simulink model "exp2_obstavoid"  (R2022a)
settings: Solver=VariableStepAuto  StartTime=0.0  StopTime=20.0  RelTol=1e-3
libraries: slpidlib x3, slctrlblks x1
settings Model: Creator=Utente  LastModifiedBy=Utente

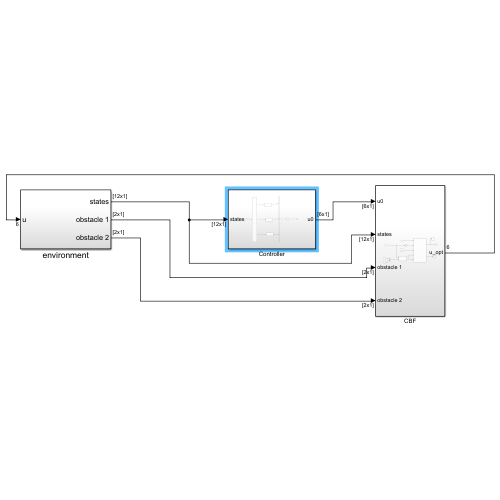
[thumbnail: Simulink's stored preview of the top-level diagram]
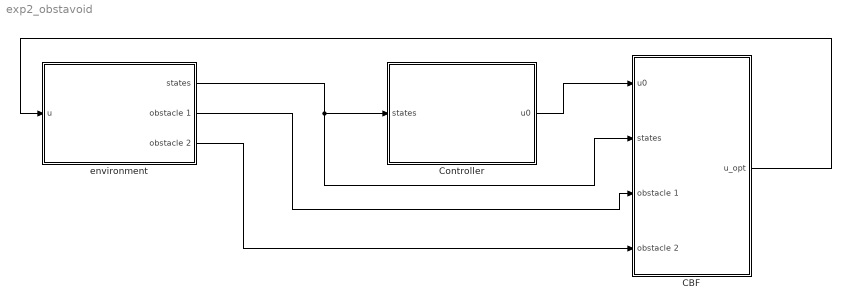
== system exp2_obstavoid ==
  CBF : Subsystem
  Controller : Subsystem
  environment : Subsystem
  wires:
  Controller/1(u0) -> CBF/1(u0)
  environment/1(states) -> CBF/2(states), Controller/1(states)
  CBF/1(u_opt) -> environment/1(u)
  environment/2(obstacle 1) -> CBF/3(obstacle 1)
  environment/3(obstacle 2) -> CBF/4(obstacle 2)

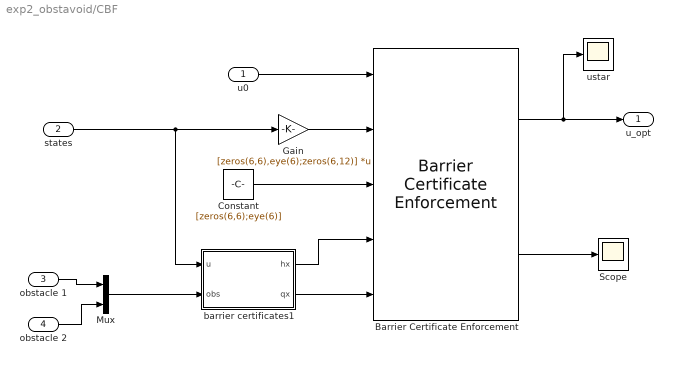
== system exp2_obstavoid/CBF ==
  u0 : Inport
  states : Inport  Port=2
  obstacle 1 : Inport  Port=3
  obstacle 2 : Inport  Port=4
  Barrier Certificate Enforcement : slctrlblks/Barrier Certificate Enforcement  nx=12  nu=6  nc=9  gamma=0.05  beta=3  external_umax=off  external_umin=off  Ts=0.1  maxiter=200  tol=1e-6  output_exitflag=on
      settings: SourceProductBaseCode=SD
  Constant : Constant  Value=[zeros(6,6);eye(6)]
  Gain : Gain  Gain=[zeros(6,6),eye(6);zeros(6,12)]  Multiplication=Matrix(K*u)
  Mux : Mux  Inputs=2
  Scope : Scope
  barrier certificates1 : MATLAB Function  TreatAsAtomicUnit=on
  ustar : Scope
  u_opt : Outport
  wires:
  Barrier Certificate Enforcement/2 -> Scope/1
  Constant/1 -> Barrier Certificate Enforcement/3
  u0/1 -> Barrier Certificate Enforcement/1
  Gain/1 -> Barrier Certificate Enforcement/2
  states/1 -> barrier certificates1/1(u), Gain/1
  Barrier Certificate Enforcement/1 -> ustar/1, u_opt/1
  barrier certificates1/1(hx) -> Barrier Certificate Enforcement/4
  barrier certificates1/2(qx) -> Barrier Certificate Enforcement/5
  obstacle 2/1 -> Mux/2
  obstacle 1/1 -> Mux/1
  Mux/1 -> barrier certificates1/2(obs)

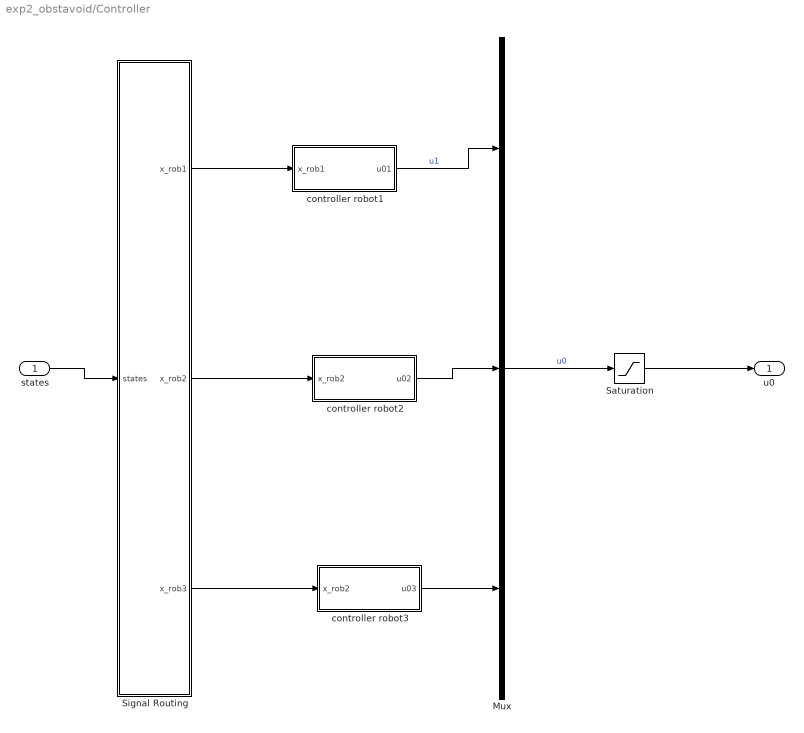
== system exp2_obstavoid/Controller ==
  states : Inport
  Mux : Mux  Inputs=3
  Saturation : Saturate  UpperLimit=10  LowerLimit=-10
  Signal Routing : MATLAB Function  TreatAsAtomicUnit=on
  controller robot1 : Subsystem
  controller robot2 : Subsystem
  controller robot3 : Subsystem
  u0 : Outport
  wires:
  states/1 -> Signal Routing/1(states)
  Signal Routing/1(x_rob1) -> controller robot1/1(x_rob1)
  Signal Routing/2(x_rob2) -> controller robot2/1(x_rob2)
  Signal Routing/3(x_rob3) -> controller robot3/1(x_rob2)
  controller robot1/1(u01) -> Mux/1  "u1"
  controller robot2/1(u02) -> Mux/2
  controller robot3/1(u03) -> Mux/3
  Mux/1 -> Saturation/1  "u0"
  Saturation/1 -> u0/1

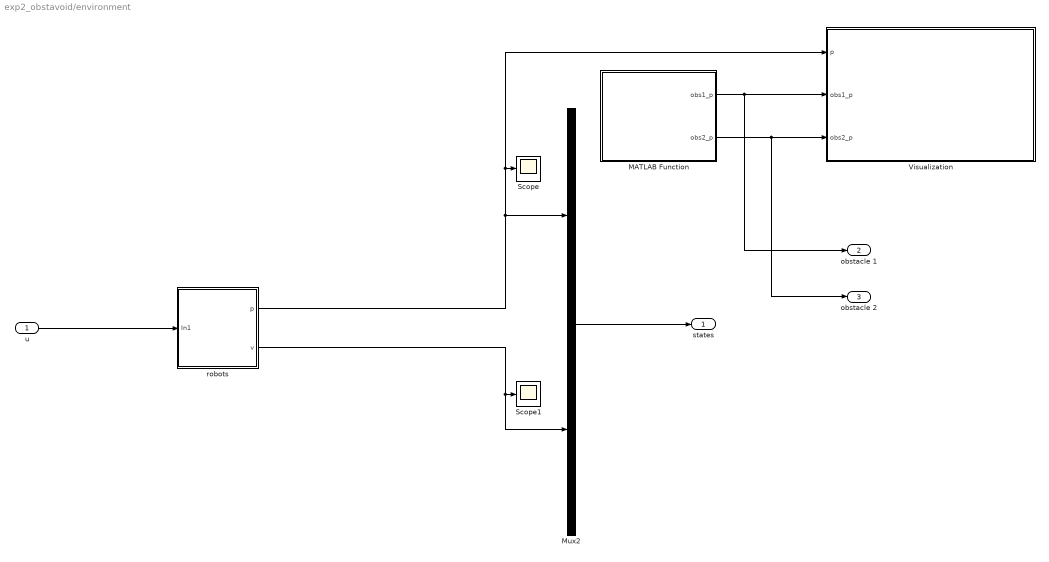
== system exp2_obstavoid/environment ==
  u : Inport
  MATLAB Function : MATLAB Function  TreatAsAtomicUnit=on
  Mux2 : Mux  Inputs=2
  Scope : Scope
  Scope1 : Scope
  Visualization : Subsystem
  robots : Subsystem
  states : Outport
  obstacle 1 : Outport  Port=2
  obstacle 2 : Outport  Port=3
  wires:
  Mux2/1 -> states/1
  robots/2(v) -> Mux2/2, Scope1/1
  robots/1(p) -> Scope/1, Visualization/1(p), Mux2/1
  u/1 -> robots/1(In1)
  MATLAB Function/1(obs1_p) -> obstacle 1/1, Visualization/2(obs1_p)
  MATLAB Function/2(obs2_p) -> obstacle 2/1, Visualization/3(obs2_p)

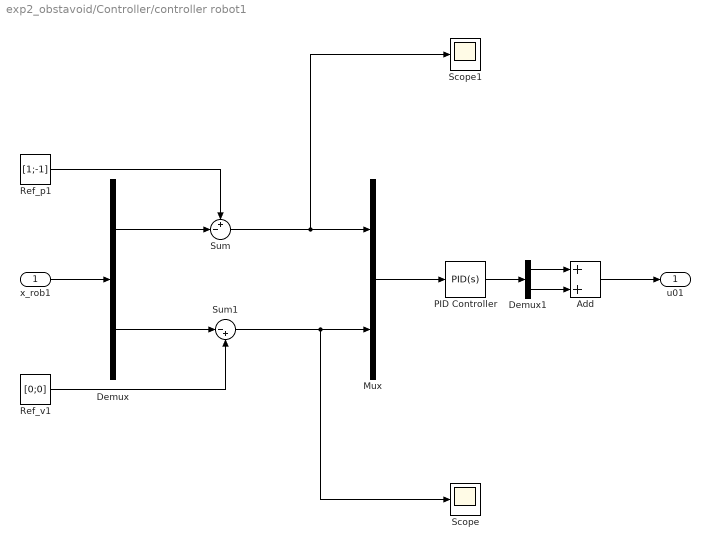
== system exp2_obstavoid/Controller/controller robot1 ==
  x_rob1 : Inport
  Add : Sum
  Demux : Demux  Outputs=2
  Demux1 : Demux  Outputs=2
  Mux : Mux  Inputs=2
  PID Controller : slpidlib/PID Controller  Controller=PID  Form=Parallel  TimeDomain=Continuous-time  UseExternalTs=off  SampleTime=-1  IntegratorMethod=Forward Euler  FilterMethod=Forward Euler  ControllerParametersSource=internal  P=5  I=0  UseKiTs=off  D=0  N=100  UseFilter=on  TunerSelectOption=Transfer Function Based (PID Tuner App)  InitialConditionSource=internal  InitialConditionForIntegrator=0  InitialConditionForFilter=0  DifferentiatorICPrevScaledInput=0  ExternalReset=none  TrackingMode=off  Kt=1  LimitOutput=off  SatLimitsSource=internal  UpperSaturationLimit=inf  LowerSaturationLimit=-inf  LinearizeAsGain=on  AntiWindupMode=none  Kb=1  POutMin=[]  POutMax=[]  IOutMin=[]  IOutMax=[]  DOutMin=[]  DOutMax=[]  NOutMin=[]  NOutMax=[]  SumOutMin=[]  SumOutMax=[]  SaturationOutMin=[]  SaturationOutMax=[]  PParamMin=[]  PParamMax=[]  IParamMin=[]  IParamMax=[]  DParamMin=[]  DParamMax=[]  NParamMin=[]  NParamMax=[]  KbParamMin=[]  KbParamMax=[]  KtParamMin=[]  KtParamMax=[]  KbOutMin=[]  KbOutMax=[]  KtOutMin=[]  KtOutMax=[]  IntegratorOutMin=[]  IntegratorOutMax=[]  FilterOutMin=[]  FilterOutMax=[]  SumI1OutMin=[]  SumI1OutMax=[]  SumI2OutMin=[]  SumI2OutMax=[]  SumI3OutMin=[]  SumI3OutMax=[]  SumI4OutMin=[]  SumI4OutMax=[]  SumDOutMin=[]  SumDOutMax=[]  DifferentiatorOutMin=[]  DifferentiatorOutMax=[]  FilterDiffOutCoefMin=[]  FilterDiffOutCoefMax=[]  ReciprocalOutMin=[]  ReciprocalOutMax=[]  SumDenOutMin=[]  SumDenOutMax=[]  SumNumOutMin=[]  SumNumOutMax=[]  DivideOutMin=[]  DivideOutMax=[]  UdiffTsProdOutMin=[]  UdiffTsProdOutMax=[]  NTsProdOutMin=[]  NTsProdOutMax=[]  UintegralTsProdOutMin=[]  UintegralTsProdOutMax=[]  UngainTsProdOutMin=[]  UngainTsProdOutMax=[]  IntegratorContinuousStateAttributes=''  IntegratorStateMustResolveToSignalObject=off  IntegratorRTWStateStorageClass=Auto  FilterContinuousStateAttributes=''  FilterStateMustResolveToSignalObject=off  FilterRTWStateStorageClass=Auto  ParallelPVariant=InternalParameters  IdealPVariant=Disabled  IVariant=InternalParameters  DVariant=InternalParameters  IntegratorVariant=Continuous  SatVariant=Disabled  AWVariant=Passthrough  PCopyVariant=Disabled  TRVariant=Disabled  FdbkBlocksVariant=Forward  IdealPFdbkVariant=Disabled  SatFdbkVariant=Disabled  DerivativeFilterVariant=ContFilter  NVariant=InternalParameters  NCopyVariant=Disabled  FilterICVariant=InternalICsFilter  IntegratorICVariant=InternalICs  ExternalResetVariant=Disabled  TRSumVariant=Passthrough  SumFdbkVariant=Disabled  SumVariant=Sum_PID  TsampFilterVariant=InternalTs  TsampNgainVariant=Passthrough  TsampIntegralVariant=Passthrough  ExternalSaturationOutDataTypeStr=Inherit: Same as second input  aMode=0
  Ref_p1 : Constant  Value=[1;-1]  VectorParams1D=off
  Ref_v1 : Constant  Value=[0;0]  VectorParams1D=off
  Scope : Scope
  Scope1 : Scope
  Sum : Sum  Inputs=+-|
  Sum1 : Sum  Inputs=|-+
  u01 : Outport
  wires:
  x_rob1/1 -> Demux/1
  Demux/1 -> Sum/2
  Ref_p1/1 -> Sum/1
  Demux/2 -> Sum1/1
  Ref_v1/1 -> Sum1/2
  Sum/1 -> Mux/1, Scope1/1
  Sum1/1 -> Mux/2, Scope/1
  Mux/1 -> PID Controller/1
  PID Controller/1 -> Demux1/1
  Demux1/2 -> Add/2
  Demux1/1 -> Add/1
  Add/1 -> u01/1

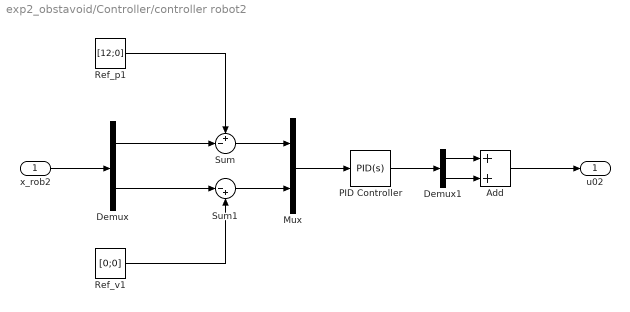
== system exp2_obstavoid/Controller/controller robot2 ==
  x_rob2 : Inport
  Add : Sum
  Demux : Demux  Outputs=2
  Demux1 : Demux  Outputs=2
  Mux : Mux  Inputs=2
  PID Controller : slpidlib/PID Controller  Controller=PID  Form=Parallel  TimeDomain=Continuous-time  UseExternalTs=off  SampleTime=-1  IntegratorMethod=Forward Euler  FilterMethod=Forward Euler  ControllerParametersSource=internal  P=5  I=0  UseKiTs=off  D=0  N=100  UseFilter=on  TunerSelectOption=Transfer Function Based (PID Tuner App)  InitialConditionSource=internal  InitialConditionForIntegrator=0  InitialConditionForFilter=0  DifferentiatorICPrevScaledInput=0  ExternalReset=none  TrackingMode=off  Kt=1  LimitOutput=off  SatLimitsSource=internal  UpperSaturationLimit=inf  LowerSaturationLimit=-inf  LinearizeAsGain=on  AntiWindupMode=none  Kb=1  POutMin=[]  POutMax=[]  IOutMin=[]  IOutMax=[]  DOutMin=[]  DOutMax=[]  NOutMin=[]  NOutMax=[]  SumOutMin=[]  SumOutMax=[]  SaturationOutMin=[]  SaturationOutMax=[]  PParamMin=[]  PParamMax=[]  IParamMin=[]  IParamMax=[]  DParamMin=[]  DParamMax=[]  NParamMin=[]  NParamMax=[]  KbParamMin=[]  KbParamMax=[]  KtParamMin=[]  KtParamMax=[]  KbOutMin=[]  KbOutMax=[]  KtOutMin=[]  KtOutMax=[]  IntegratorOutMin=[]  IntegratorOutMax=[]  FilterOutMin=[]  FilterOutMax=[]  SumI1OutMin=[]  SumI1OutMax=[]  SumI2OutMin=[]  SumI2OutMax=[]  SumI3OutMin=[]  SumI3OutMax=[]  SumI4OutMin=[]  SumI4OutMax=[]  SumDOutMin=[]  SumDOutMax=[]  DifferentiatorOutMin=[]  DifferentiatorOutMax=[]  FilterDiffOutCoefMin=[]  FilterDiffOutCoefMax=[]  ReciprocalOutMin=[]  ReciprocalOutMax=[]  SumDenOutMin=[]  SumDenOutMax=[]  SumNumOutMin=[]  SumNumOutMax=[]  DivideOutMin=[]  DivideOutMax=[]  UdiffTsProdOutMin=[]  UdiffTsProdOutMax=[]  NTsProdOutMin=[]  NTsProdOutMax=[]  UintegralTsProdOutMin=[]  UintegralTsProdOutMax=[]  UngainTsProdOutMin=[]  UngainTsProdOutMax=[]  IntegratorContinuousStateAttributes=''  IntegratorStateMustResolveToSignalObject=off  IntegratorRTWStateStorageClass=Auto  FilterContinuousStateAttributes=''  FilterStateMustResolveToSignalObject=off  FilterRTWStateStorageClass=Auto  ParallelPVariant=InternalParameters  IdealPVariant=Disabled  IVariant=InternalParameters  DVariant=InternalParameters  IntegratorVariant=Continuous  SatVariant=Disabled  AWVariant=Passthrough  PCopyVariant=Disabled  TRVariant=Disabled  FdbkBlocksVariant=Forward  IdealPFdbkVariant=Disabled  SatFdbkVariant=Disabled  DerivativeFilterVariant=ContFilter  NVariant=InternalParameters  NCopyVariant=Disabled  FilterICVariant=InternalICsFilter  IntegratorICVariant=InternalICs  ExternalResetVariant=Disabled  TRSumVariant=Passthrough  SumFdbkVariant=Disabled  SumVariant=Sum_PID  TsampFilterVariant=InternalTs  TsampNgainVariant=Passthrough  TsampIntegralVariant=Passthrough  ExternalSaturationOutDataTypeStr=Inherit: Same as second input  aMode=0
  Ref_p1 : Constant  Value=[12;0]  VectorParams1D=off
  Ref_v1 : Constant  Value=[0;0]  VectorParams1D=off
  Sum : Sum  Inputs=+-|
  Sum1 : Sum  Inputs=|-+
  u02 : Outport
  wires:
  x_rob2/1 -> Demux/1
  Demux/1 -> Sum/2
  Ref_p1/1 -> Sum/1
  Demux/2 -> Sum1/1
  Ref_v1/1 -> Sum1/2
  Add/1 -> u02/1
  Demux1/2 -> Add/2
  Mux/1 -> PID Controller/1
  Sum/1 -> Mux/1
  Sum1/1 -> Mux/2
  PID Controller/1 -> Demux1/1
  Demux1/1 -> Add/1

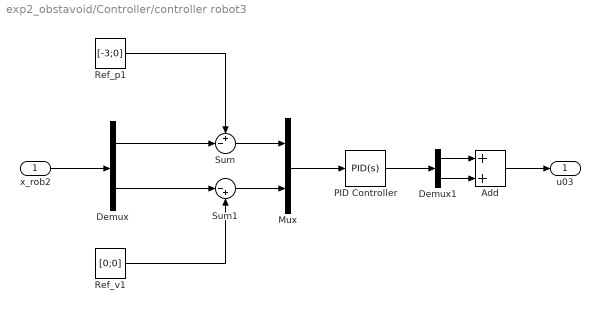
== system exp2_obstavoid/Controller/controller robot3 ==
  x_rob2 : Inport
  Add : Sum
  Demux : Demux  Outputs=2
  Demux1 : Demux  Outputs=2
  Mux : Mux  Inputs=2
  PID Controller : slpidlib/PID Controller  Controller=PID  Form=Parallel  TimeDomain=Continuous-time  UseExternalTs=off  SampleTime=-1  IntegratorMethod=Forward Euler  FilterMethod=Forward Euler  ControllerParametersSource=internal  P=5  I=0  UseKiTs=off  D=0  N=100  UseFilter=on  TunerSelectOption=Transfer Function Based (PID Tuner App)  InitialConditionSource=internal  InitialConditionForIntegrator=0  InitialConditionForFilter=0  DifferentiatorICPrevScaledInput=0  ExternalReset=none  TrackingMode=off  Kt=1  LimitOutput=off  SatLimitsSource=internal  UpperSaturationLimit=inf  LowerSaturationLimit=-inf  LinearizeAsGain=on  AntiWindupMode=none  Kb=1  POutMin=[]  POutMax=[]  IOutMin=[]  IOutMax=[]  DOutMin=[]  DOutMax=[]  NOutMin=[]  NOutMax=[]  SumOutMin=[]  SumOutMax=[]  SaturationOutMin=[]  SaturationOutMax=[]  PParamMin=[]  PParamMax=[]  IParamMin=[]  IParamMax=[]  DParamMin=[]  DParamMax=[]  NParamMin=[]  NParamMax=[]  KbParamMin=[]  KbParamMax=[]  KtParamMin=[]  KtParamMax=[]  KbOutMin=[]  KbOutMax=[]  KtOutMin=[]  KtOutMax=[]  IntegratorOutMin=[]  IntegratorOutMax=[]  FilterOutMin=[]  FilterOutMax=[]  SumI1OutMin=[]  SumI1OutMax=[]  SumI2OutMin=[]  SumI2OutMax=[]  SumI3OutMin=[]  SumI3OutMax=[]  SumI4OutMin=[]  SumI4OutMax=[]  SumDOutMin=[]  SumDOutMax=[]  DifferentiatorOutMin=[]  DifferentiatorOutMax=[]  FilterDiffOutCoefMin=[]  FilterDiffOutCoefMax=[]  ReciprocalOutMin=[]  ReciprocalOutMax=[]  SumDenOutMin=[]  SumDenOutMax=[]  SumNumOutMin=[]  SumNumOutMax=[]  DivideOutMin=[]  DivideOutMax=[]  UdiffTsProdOutMin=[]  UdiffTsProdOutMax=[]  NTsProdOutMin=[]  NTsProdOutMax=[]  UintegralTsProdOutMin=[]  UintegralTsProdOutMax=[]  UngainTsProdOutMin=[]  UngainTsProdOutMax=[]  IntegratorContinuousStateAttributes=''  IntegratorStateMustResolveToSignalObject=off  IntegratorRTWStateStorageClass=Auto  FilterContinuousStateAttributes=''  FilterStateMustResolveToSignalObject=off  FilterRTWStateStorageClass=Auto  ParallelPVariant=InternalParameters  IdealPVariant=Disabled  IVariant=InternalParameters  DVariant=InternalParameters  IntegratorVariant=Continuous  SatVariant=Disabled  AWVariant=Passthrough  PCopyVariant=Disabled  TRVariant=Disabled  FdbkBlocksVariant=Forward  IdealPFdbkVariant=Disabled  SatFdbkVariant=Disabled  DerivativeFilterVariant=ContFilter  NVariant=InternalParameters  NCopyVariant=Disabled  FilterICVariant=InternalICsFilter  IntegratorICVariant=InternalICs  ExternalResetVariant=Disabled  TRSumVariant=Passthrough  SumFdbkVariant=Disabled  SumVariant=Sum_PID  TsampFilterVariant=InternalTs  TsampNgainVariant=Passthrough  TsampIntegralVariant=Passthrough  ExternalSaturationOutDataTypeStr=Inherit: Same as second input  aMode=0
  Ref_p1 : Constant  Value=[-3;0]  VectorParams1D=off
  Ref_v1 : Constant  Value=[0;0]  VectorParams1D=off
  Sum : Sum  Inputs=+-|
  Sum1 : Sum  Inputs=|-+
  u03 : Outport
  wires:
  x_rob2/1 -> Demux/1
  Demux/1 -> Sum/2
  Ref_p1/1 -> Sum/1
  Demux/2 -> Sum1/1
  Ref_v1/1 -> Sum1/2
  Add/1 -> u03/1
  Demux1/2 -> Add/2
  Demux1/1 -> Add/1
  Sum1/1 -> Mux/2
  Sum/1 -> Mux/1
  PID Controller/1 -> Demux1/1
  Mux/1 -> PID Controller/1

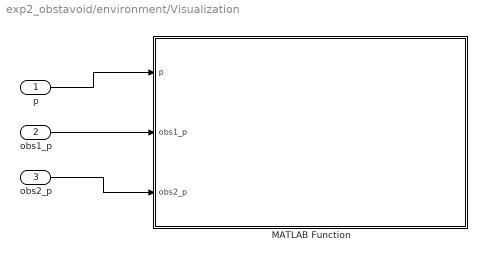
== system exp2_obstavoid/environment/Visualization ==
  p : Inport
  obs1_p : Inport  Port=2
  obs2_p : Inport  Port=3
  MATLAB Function : MATLAB Function  TreatAsAtomicUnit=on
  wires:
  p/1 -> MATLAB Function/1(p)
  obs1_p/1 -> MATLAB Function/2(obs1_p)
  obs2_p/1 -> MATLAB Function/3(obs2_p)

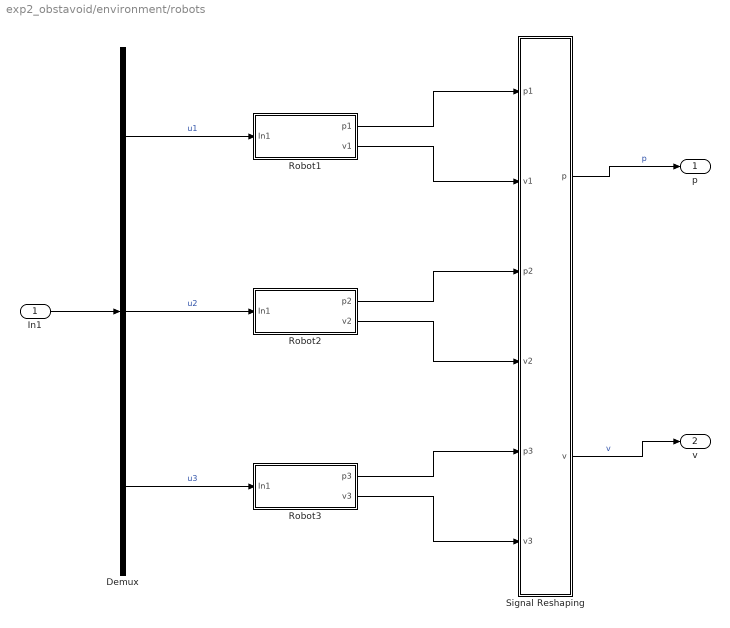
== system exp2_obstavoid/environment/robots ==
  In1 : Inport
  Demux : Demux  Outputs=3
  Robot1 : Subsystem
  Robot2 : Subsystem
  Robot3 : Subsystem
  Signal Reshaping : MATLAB Function  TreatAsAtomicUnit=on
  p : Outport
  v : Outport  Port=2
  wires:
  Robot2/2(v2) -> Signal Reshaping/4(v2)
  Robot3/2(v3) -> Signal Reshaping/6(v3)
  Robot2/1(p2) -> Signal Reshaping/3(p2)
  Robot1/1(p1) -> Signal Reshaping/1(p1)
  Robot3/1(p3) -> Signal Reshaping/5(p3)
  Robot1/2(v1) -> Signal Reshaping/2(v1)
  In1/1 -> Demux/1
  Demux/1 -> Robot1/1(In1)  "u1"
  Demux/2 -> Robot2/1(In1)  "u2"
  Demux/3 -> Robot3/1(In1)  "u3"
  Signal Reshaping/2(v) -> v/1  "v"
  Signal Reshaping/1(p) -> p/1  "p"

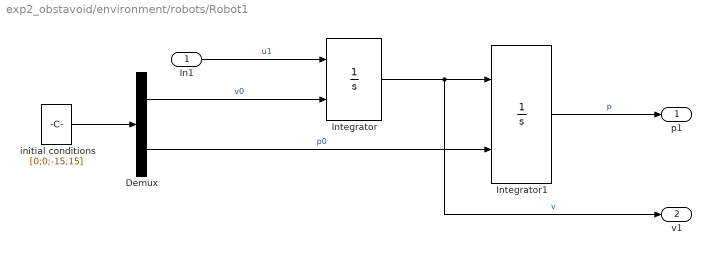
== system exp2_obstavoid/environment/robots/Robot1 ==
  In1 : Inport
  Demux : Demux  Outputs=2
  Integrator : Integrator  InitialConditionSource=external  LimitOutput=on  UpperSaturationLimit=2  LowerSaturationLimit=-2
  Integrator1 : Integrator  InitialConditionSource=external
  initial conditions : Constant  Value=[0;0;-15;15]  VectorParams1D=off
  p1 : Outport
  v1 : Outport  Port=2
  wires:
  initial conditions/1 -> Demux/1
  In1/1 -> Integrator/1  "u1"
  Demux/1 -> Integrator/2  "v0"
  Integrator/1 -> Integrator1/1, v1/1  "v"
  Demux/2 -> Integrator1/2  "p0"
  Integrator1/1 -> p1/1  "p"

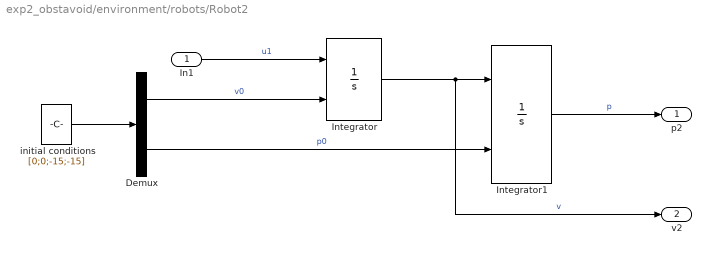
== system exp2_obstavoid/environment/robots/Robot2 ==
  In1 : Inport
  Demux : Demux  Outputs=2
  Integrator : Integrator  InitialConditionSource=external  LimitOutput=on  UpperSaturationLimit=2  LowerSaturationLimit=-2
  Integrator1 : Integrator  InitialConditionSource=external
  initial conditions : Constant  Value=[0;0;-15;-15]  VectorParams1D=off
  p2 : Outport
  v2 : Outport  Port=2
  wires:
  initial conditions/1 -> Demux/1
  In1/1 -> Integrator/1  "u1"
  Demux/1 -> Integrator/2  "v0"
  Integrator/1 -> v2/1, Integrator1/1  "v"
  Demux/2 -> Integrator1/2  "p0"
  Integrator1/1 -> p2/1  "p"

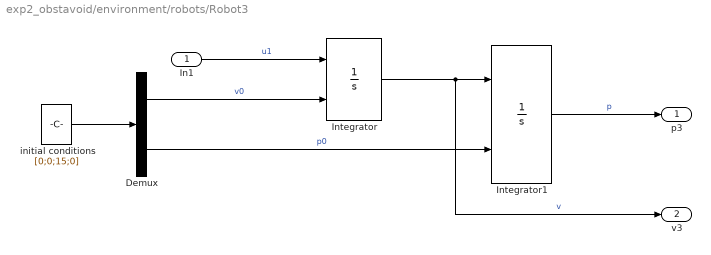
== system exp2_obstavoid/environment/robots/Robot3 ==
  In1 : Inport
  Demux : Demux  Outputs=2
  Integrator : Integrator  InitialConditionSource=external  LimitOutput=on  UpperSaturationLimit=2  LowerSaturationLimit=-2
  Integrator1 : Integrator  InitialConditionSource=external
  initial conditions : Constant  Value=[0;0;15;0]  VectorParams1D=off
  p3 : Outport
  v3 : Outport  Port=2
  wires:
  initial conditions/1 -> Demux/1
  In1/1 -> Integrator/1  "u1"
  Demux/1 -> Integrator/2  "v0"
  Integrator/1 -> v3/1, Integrator1/1  "v"
  Demux/2 -> Integrator1/2  "p0"
  Integrator1/1 -> p3/1  "p"

== matlab function exp2_obstavoid/Controller/Signal Routing ==
  data: states input; x_rob1 output; x_rob2 output; x_rob3 output
function [x_rob1, x_rob2, x_rob3] = fcn(states)


x_rob1 = [states(1); states(2); states(7); states(8)];
x_rob2 = [states(3); states(4); states(9); states(10)];
x_rob3 = [states(5); states(6); states(11); states(12)];

== matlab function exp2_obstavoid/environment/robots/Signal Reshaping ==
  data: p1 input; p output; v1 input; p2 input; v2 input; p3 input; v3 input; v output
function [p,v] = fcn(p1,v1,p2,v2,p3,v3)

p = [p1;p2;p3];
v = [v1;v2;v3];

== matlab function exp2_obstavoid/environment/Visualization/MATLAB Function ==
  data: p input; obs1_p input; obs2_p input
function fcn(p, obs1_p, obs2_p)
Nrobots = 3;                    % number of robots in simulation
RobotRadius = 1;                % desired robot radius
Nobstacles = 2;
colors = {"red", "blue", "green", "cyan", "magenta", "black", "yellow", "#EDB120"}; %colors

x_robots = [p(1); p(3); p(5)];
y_robots = [p(2); p(4); p(6)];

StartPos = [x_robots y_robots];




for i=1:Nrobots
    
    % create the ith robot 
    pos = [StartPos(i,:)-RobotRadius 2*RobotRadius 2*RobotRadius]; %position of the robot by considering its radius
    r = rectangle('Position', pos, 'Curvature',[1 1], 'FaceColor', colors{i}, 'Edgecolor','none'); %graph of the robot as it were a kind of circle, for simplicity
    
    axis([-30 30 -30 30]) %axis of the graph: x axis from -30 to 30, the same for y
    title('Robots simulation');
    figure(1); hold on;
    %pause(0.5); 
    
  
end

%clf %uncomment this if you want to see only the robots, comment this if
%you want to see also the robots' trajectories

obs1_p = obs1_p.';
obs2_p = obs2_p.';
obs_radius = 2;
pos_obs1 = [obs1_p(1,:)-obs_radius 2*obs_radius 2*obs_radius];
pos_obs2 = [obs2_p(1,:)-obs_radius 2*obs_radius 2*obs_radius];

r_obs1 = rectangle('Position', pos_obs1, 'Curvature',[1 1], 'FaceColor', colors{i+1}, 'Edgecolor','none');
r_obs2 = rectangle('Position', pos_obs2, 'Curvature',[1 1], 'FaceColor', colors{i+2}, 'Edgecolor','none');

== matlab function exp2_obstavoid/environment/MATLAB Function ==
  data: obs1_p output; obs2_p output
function [obs1_p, obs2_p] = obstacles()

px_obs1 = 6;
py_obs1 = 2;
obs1_p = [px_obs1; py_obs1];

px_obs2 = -10;
py_obs2 = -8;
obs2_p = [px_obs2; py_obs2];

== matlab function exp2_obstavoid/CBF/barrier certificates1 ==
  data: u input; hx output; qx output; obs input
function [hx,qx] = fcn(u,obs)


[hx,qx] = CBFthreeRobotsandStatObs(u,obs);
